simulink model "DISCON_NREL5MW_update"  (R2020b)
settings: Solver=FixedStepDiscrete  StartTime=0.0  StopTime=inf  FixedStep=Control.DT  RelTol=1e-3
values from neighbouring files (symbols this model uses):
  Gd_Fwave = c2d(Sys{OperatingPoint}('omega_r','F_{hydro}'),Control.TimeStep,'tustin')    [ControlParams_NREL5MW.m]
  Gd_Mwave = c2d(Sys{OperatingPoint}('omega_r','M_{hydro}'),Control.TimeStep,'tustin')    [ControlParams_NREL5MW.m]
  InvGp = inv(Gp)    [ControlParams_NREL5MW.m]
  Kff_gain = 0.3    [InitCompDISCON.m]
undefined symbols (not defined in the file or in its folder): CertificationSettings, Control, DelTFd, DiscIntNeverNeededParam, Drivetrain, Freq_Mixing, P_InitAngle
settings Model: Creator=evansolingen  LastModifiedBy=ahegazy
settings DataIOCC: LimitDataPoints=on  SaveFormat=Array  SignalLoggingSaveFormat=ModelDataLogs  SaveOutput=off  SignalLogging=off  SaveTime=off  ReturnWorkspaceOutputs=off
settings OptimizationCC: ExpressionDepthLimit=2147483647  LifeSpan=inf
settings DebuggingCC: UnderspecifiedInitializationDetection=Classic  MergeDetectMultiDrivingBlocksExec=none  SolverPrmCheckMsg=warning  MultiTaskDSMMsg=warning  MultiTaskCondExecSysMsg=none  FcnCallInpInsideContextMsg=warning  AllowSymbolicDim=off  StateNameClashWarn=warning  SFUnexpectedBacktrackingDiag=warning  SFNoUnconditionalDefaultTransitionDiag=warning  SFExecutionAtInitializationDiag=none  ArithmeticOperatorsInVariantConditions=warning
settings HardwareCC: ProdBitPerPointer=32  ProdBitPerSizeT=32  ProdBitPerPtrDiffT=32  ProdLargestAtomicFloat=None  ProdIntDivRoundTo=Undefined  ProdEndianess=Unspecified  ProdWordSize=32  ProdHWDeviceType=32-bit Generic
settings ModelReferenceCC: UpdateModelReferenceTargets=Force  PropagateSignalLabelsOutOfModel=off
settings SFSimCC: SimUseLocalCustomCode=off  SimParseCustomCode=off  CustomCodeUndefinedFunction=UseInterfaceOnly
settings RTWCC: Description=DISCON DLL Target (for use with GH BLADED)  SystemTargetFile=discon.tlc  TemplateMakefile=discon_vc.tmf  RTWUseLocalCustomCode=off
settings CodeAppCC: StateflowObjectComments=on
settings GRTTargetCC: TargetLangStandard=C89/C90 (ANSI)  CombineOutputUpdateFcns=off  GRTInterface=on  UseToolchainInfoCompliant=off  ExtModeMexFile=noextcomm
settings ConfigComp: CovMetricSettings=dw  CovSaveCumulativeToWorkspaceVar=on  CovSaveSingleToWorkspaceVar=on  CovExternalEMLEnable=off

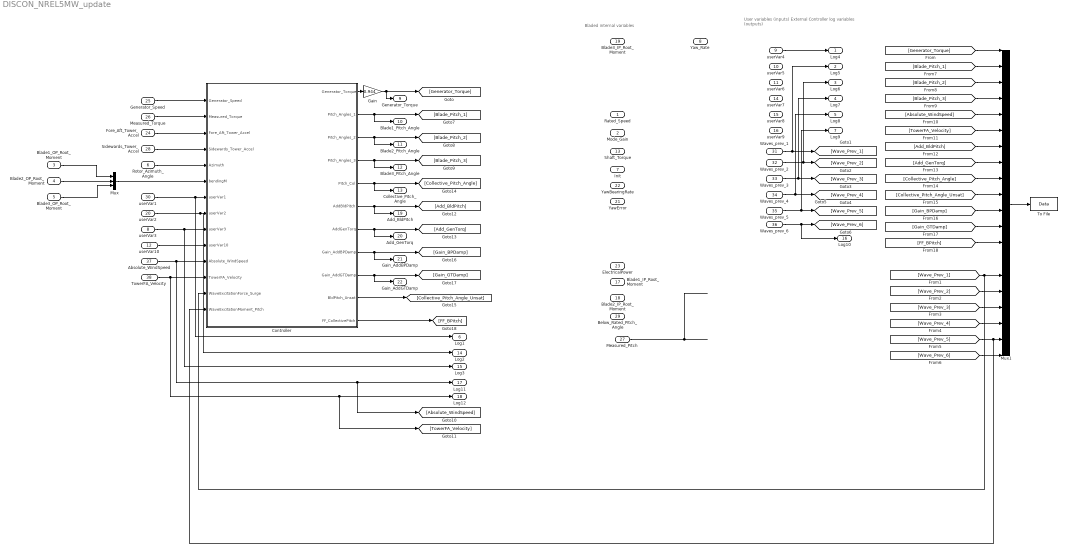
== system DISCON_NREL5MW_update ==
  note: Bladed internal variables
  note: User variables (inputs)
      | External Controller log variables (outputs)
  Rated_Speed : Inport  PortDimensions=1
  Mode_Gain : Inport  Port=2  PortDimensions=1
  Blade1_OP_Root_Moment : Inport  Port=3  PortDimensions=1
  Blade2_OP_Root_Moment : Inport  Port=4  PortDimensions=1
  Blade3_OP_Root_Moment : Inport  Port=5  PortDimensions=1
  Rotor_Azimuth_Angle : Inport  Port=6  PortDimensions=1
  Init : Inport  Port=7  PortDimensions=1
  userVar3 : Inport  Port=8  PortDimensions=1
  userVar4 : Inport  Port=9  PortDimensions=1
  userVar5 : Inport  Port=10  PortDimensions=1
  userVar6 : Inport  Port=11  PortDimensions=1
  userVar10 : Inport  Port=12  PortDimensions=1
  Shaft_Torque : Inport  Port=13  PortDimensions=1
  userVar7 : Inport  Port=14  PortDimensions=1
  userVar8 : Inport  Port=15  PortDimensions=1
  userVar9 : Inport  Port=16  PortDimensions=1
  Blade1_IP_Root_Moment : Inport  Port=17  PortDimensions=1
  Blade2_IP_Root_Moment : Inport  Port=18  PortDimensions=1
  Blade3_IP_Root_Moment : Inport  Port=19  PortDimensions=1
  userVar2 : Inport  Port=20  PortDimensions=1
  YawError : Inport  Port=21  PortDimensions=1
  YawBearingRate : Inport  Port=22  PortDimensions=1
  ElectricalPower : Inport  Port=23  PortDimensions=1
  Fore_Aft_Tower_Accel : Inport  Port=24  PortDimensions=1
  Generator_Speed : Inport  Port=25  PortDimensions=1
  Measured_Torque : Inport  Port=26  PortDimensions=1
  Measured_Pitch : Inport  Port=27  PortDimensions=1
  Sidewards_Tower_Accel : Inport  Port=28  PortDimensions=1
  Below_Rated_Pitch_Angle : Inport  Port=29  PortDimensions=1
  userVar1 : Inport  Port=30  PortDimensions=1
  Waves_prev_1 : Inport  Port=31  PortDimensions=1
  Waves_prev_2 : Inport  Port=32  PortDimensions=1
  Waves_prev_3 : Inport  Port=33  PortDimensions=1
  Waves_prev_4 : Inport  Port=34  PortDimensions=1
  Waves_prev_5 : Inport  Port=35  PortDimensions=1
  Waves_prev_6 : Inport  Port=36  PortDimensions=1
  Absolute_WindSpeed : Inport  Port=37  PortDimensions=1
  TowerFA_Velocity : Inport  Port=38  PortDimensions=1
  Controller : Subsystem
  Gain : Gain  Gain=0.944
  Mux : Mux  Inputs=3
  Mux1 : Mux  Inputs=20
  To File : ToFile  Filename=Data  MatrixName=Data
  Log4 : Outport  PortDimensions=1  VectorParamsAs1DForOutWhenUnconnected=off
  Log5 : Outport  Port=2  PortDimensions=1  VectorParamsAs1DForOutWhenUnconnected=off
  Log6 : Outport  Port=3  PortDimensions=1  VectorParamsAs1DForOutWhenUnconnected=off
  Log7 : Outport  Port=4  PortDimensions=1  VectorParamsAs1DForOutWhenUnconnected=off
  Log8 : Outport  Port=5  PortDimensions=1  VectorParamsAs1DForOutWhenUnconnected=off
  Log1 : Outport  Port=6  PortDimensions=1  VectorParamsAs1DForOutWhenUnconnected=off
  Log9 : Outport  Port=7  PortDimensions=1  VectorParamsAs1DForOutWhenUnconnected=off
  Yaw_Rate : Outport  Port=8  PortDimensions=1  VectorParamsAs1DForOutWhenUnconnected=off
  Generator_Torque : Outport  Port=9  PortDimensions=1  VectorParamsAs1DForOutWhenUnconnected=off
  Blade1_Pitch_Angle : Outport  Port=10  PortDimensions=1  VectorParamsAs1DForOutWhenUnconnected=off
  Blade2_Pitch_Angle : Outport  Port=11  PortDimensions=1  VectorParamsAs1DForOutWhenUnconnected=off
  Blade3_Pitch_Angle : Outport  Port=12  PortDimensions=1  VectorParamsAs1DForOutWhenUnconnected=off
  Collective_Pitch_Angle : Outport  Port=13  PortDimensions=1  VectorParamsAs1DForOutWhenUnconnected=off
  Log2 : Outport  Port=14  PortDimensions=1  VectorParamsAs1DForOutWhenUnconnected=off
  Log3 : Outport  Port=15  PortDimensions=1  VectorParamsAs1DForOutWhenUnconnected=off
  Log10 : Outport  Port=16  PortDimensions=1  VectorParamsAs1DForOutWhenUnconnected=off
  Log11 : Outport  Port=17  PortDimensions=1  VectorParamsAs1DForOutWhenUnconnected=off
  Log12 : Outport  Port=18  PortDimensions=1  VectorParamsAs1DForOutWhenUnconnected=off
  Add_BldPitch : Outport  Port=19  PortDimensions=1  VectorParamsAs1DForOutWhenUnconnected=off
  Add_GenTorq : Outport  Port=20  PortDimensions=1  VectorParamsAs1DForOutWhenUnconnected=off
  Gain_AddBPDamp : Outport  Port=21  PortDimensions=1  VectorParamsAs1DForOutWhenUnconnected=off
  Gain_AddGTDamp : Outport  Port=22  PortDimensions=1  VectorParamsAs1DForOutWhenUnconnected=off
  wires:
  Fore_Aft_Tower_Accel/1 -> Controller/3(Fore_Aft_Tower_Accel)
  Measured_Pitch/1 -> ?
  Generator_Speed/1 -> Controller/1(Generator_Speed)
  Controller/1(Generator_Torque) -> Gain/1
  userVar3/1 -> Log3/1, Controller/9(userVar3)
  userVar4/1 -> Log4/1
  Gain/1 -> [Generator_Torque], Generator_Torque/1
  Measured_Torque/1 -> Controller/2(Measured_Torque)
  Sidewards_Tower_Accel/1 -> Controller/4(Sidewards_Tower_Accel)
  Rotor_Azimuth_Angle/1 -> Controller/5(Azimuth)
  Blade1_OP_Root_Moment/1 -> Mux/1
  Blade2_OP_Root_Moment/1 -> Mux/2
  Blade3_OP_Root_Moment/1 -> Mux/3
  Mux/1 -> Controller/6(bendingM)
  Controller/2(Pitch_Angles_1) -> Blade1_Pitch_Angle/1, [Blade_Pitch_1]
  Controller/3(Pitch_Angles_2) -> Blade2_Pitch_Angle/1, [Blade_Pitch_2]
  Controller/4(Pitch_Angles_3) -> Blade3_Pitch_Angle/1, [Blade_Pitch_3]
  Controller/5(Pitch_Col) -> [Collective_Pitch_Angle], Collective_Pitch_Angle/1
  userVar1/1 -> Log1/1, Controller/7(userVar1)
  userVar2/1 -> Log2/1, Controller/8(userVar2)
  userVar10/1 -> Controller/10(userVar10)
  Mux1/1 -> To File/1
  [Generator_Torque] -> Mux1/1
  Waves_prev_1/1 -> Log5/1, [Wave_Prev_1]
  Waves_prev_2/1 -> Log6/1, [Wave_Prev_2]
  Waves_prev_3/1 -> Log7/1, [Wave_Prev_3]
  Waves_prev_4/1 -> Log8/1, [Wave_Prev_4]
  Waves_prev_5/1 -> Log9/1, [Wave_Prev_5]
  Waves_prev_6/1 -> Log10/1, [Wave_Prev_6]
  [Wave_Prev_6] -> Mux1/20
  [Wave_Prev_5] -> Controller/14(WaveExcitationMoment_Pitch), Mux1/19
  [Wave_Prev_4] -> Mux1/18
  [Wave_Prev_3] -> Mux1/17
  [Wave_Prev_2] -> Mux1/16
  [Wave_Prev_1] -> Mux1/15, Controller/13(WaveExcitationForce_Surge)
  [Blade_Pitch_1] -> Mux1/2
  [Blade_Pitch_2] -> Mux1/3
  [Blade_Pitch_3] -> Mux1/4
  TowerFA_Velocity/1 -> Controller/12(TowerFA_Velocity), [TowerFA_Velocity], Log12/1
  [Absolute_WindSpeed] -> Mux1/5
  [TowerFA_Velocity] -> Mux1/6
  [Add_BldPitch] -> Mux1/7
  [Add_GenTorq] -> Mux1/8
  Absolute_WindSpeed/1 -> [Absolute_WindSpeed], Log11/1, Controller/11(Absolute_WindSpeed)
  Controller/6(AddBldPitch) -> Add_BldPitch/1, [Add_BldPitch]
  Controller/7(AddGenTorq) -> Add_GenTorq/1, [Add_GenTorq]
  Controller/8(Gain_AddBPDamp) -> Gain_AddBPDamp/1, [Gain_BPDamp]
  Controller/9(Gain_AddGTDamp) -> Gain_AddGTDamp/1, [Gain_GTDamp]
  [Collective_Pitch_Angle] -> Mux1/9
  Controller/10(BldPitch_Unsat) -> [Collective_Pitch_Angle_Unsat]
  [Collective_Pitch_Angle_Unsat] -> Mux1/10
  [Gain_BPDamp] -> Mux1/11
  [Gain_GTDamp] -> Mux1/12
  [FF_BPitch] -> Mux1/13
  Controller/11(FF_CollectivePitch) -> [FF_BPitch]

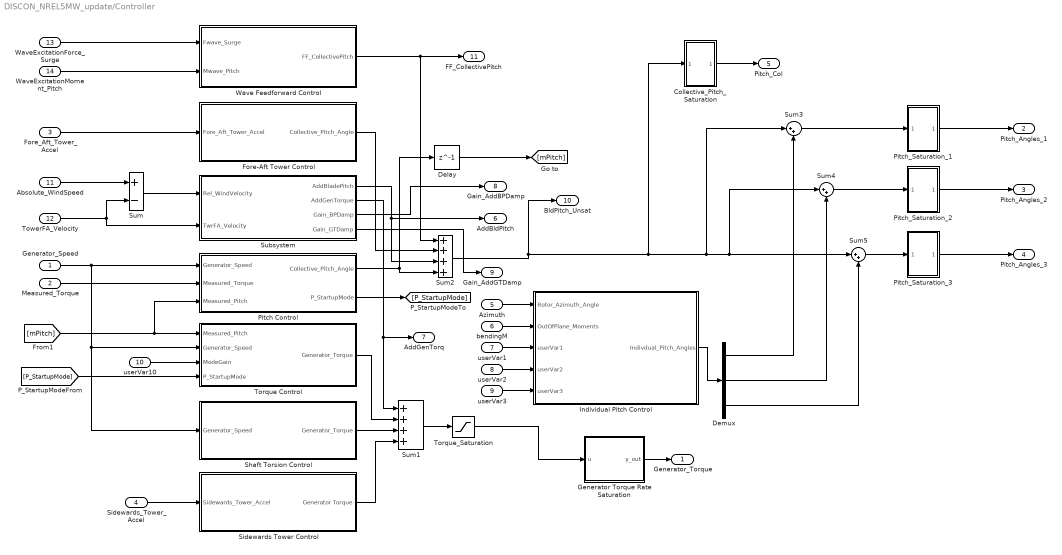
== system DISCON_NREL5MW_update/Controller ==
  Generator_Speed : Inport
  Measured_Torque : Inport  Port=2
  Fore_Aft_Tower_Accel : Inport  Port=3
  Sidewards_Tower_Accel : Inport  Port=4  PortDimensions=1
  Azimuth : Inport  Port=5  PortDimensions=1
  bendingM : Inport  Port=6
  userVar1 : Inport  Port=7  PortDimensions=1
  userVar2 : Inport  Port=8  PortDimensions=1
  userVar3 : Inport  Port=9  PortDimensions=1
  userVar10 : Inport  Port=10  PortDimensions=1
  Absolute_WindSpeed : Inport  Port=11  PortDimensions=1
  TowerFA_Velocity : Inport  Port=12  PortDimensions=1
  WaveExcitationForce_Surge : Inport  Port=13
  WaveExcitationMoment_Pitch : Inport  Port=14
  Collective_Pitch_Saturation : Subsystem
  Delay : Delay  DelayLength=1
  Demux : Demux  Outputs=3
  Fore-Aft Tower Control : Subsystem
  Generator Torque Rate Saturation : Subsystem
  Individual Pitch Control : Subsystem
  Pitch Control : Subsystem
  Pitch_Saturation_1 : Subsystem
  Pitch_Saturation_2 : Subsystem
  Pitch_Saturation_3 : Subsystem
  Shaft Torsion Control : Subsystem
  Sidewards Tower Control : Subsystem
  Subsystem : Subsystem
  Sum : Sum  Inputs=+-
  Sum1 : Sum  Inputs=++++
  Sum2 : Sum  Inputs=++++
  Sum3 : Sum  Inputs=|++
  Sum4 : Sum  Inputs=|++
  Sum5 : Sum  Inputs=|++
  Torque Control : Subsystem
  Torque_Saturation : Saturate  UpperLimit=Control.Torque.Limit  LowerLimit=Control.Torque.Min
  Wave Feedforward Control : Subsystem
  Generator_Torque : Outport  VectorParamsAs1DForOutWhenUnconnected=off
  Pitch_Angles_1 : Outport  Port=2  PortDimensions=1  VectorParamsAs1DForOutWhenUnconnected=off
  Pitch_Angles_2 : Outport  Port=3  PortDimensions=1  VectorParamsAs1DForOutWhenUnconnected=off
  Pitch_Angles_3 : Outport  Port=4  PortDimensions=1  VectorParamsAs1DForOutWhenUnconnected=off
  Pitch_Col : Outport  Port=5  PortDimensions=1  VectorParamsAs1DForOutWhenUnconnected=off
  AddBldPitch : Outport  Port=6  PortDimensions=1  VectorParamsAs1DForOutWhenUnconnected=off
  AddGenTorq : Outport  Port=7  PortDimensions=1  VectorParamsAs1DForOutWhenUnconnected=off
  Gain_AddBPDamp : Outport  Port=8  PortDimensions=1  VectorParamsAs1DForOutWhenUnconnected=off
  Gain_AddGTDamp : Outport  Port=9  PortDimensions=1  VectorParamsAs1DForOutWhenUnconnected=off
  BldPitch_Unsat : Outport  Port=10  PortDimensions=1  VectorParamsAs1DForOutWhenUnconnected=off
  FF_CollectivePitch : Outport  Port=11
  wires:
  Sidewards_Tower_Accel/1 -> Sidewards Tower Control/1(Sidewards_Tower_Accel)
  Fore_Aft_Tower_Accel/1 -> Fore-Aft Tower Control/1(Fore_Aft_Tower_Accel)
  Fore-Aft Tower Control/1(Collective_Pitch_Angle) -> Sum2/2
  Torque Control/1(Generator_Torque) -> Sum1/2
  Sidewards Tower Control/1(Generator Torque) -> Sum1/4
  Measured_Torque/1 -> Pitch Control/2(Measured_Torque)
  Shaft Torsion Control/1(Generator_Torque) -> Sum1/3
  userVar10/1 -> Torque Control/3(ModeGain)
  Sum1/1 -> Torque_Saturation/1
  Pitch_Saturation_1/1(y_out) -> Pitch_Angles_1/1
  Generator_Speed/1 -> Torque Control/2(Generator_Speed), Shaft Torsion Control/1(Generator_Speed), Pitch Control/1(Generator_Speed)
  [P_StartupMode] -> Torque Control/4(P_StartupMode)
  Pitch Control/2(P_StartupMode) -> [P_StartupMode]
  Pitch Control/1(Collective_Pitch_Angle) -> Delay/1, Sum2/4
  Pitch_Saturation_2/1(y_out) -> Pitch_Angles_2/1
  Pitch_Saturation_3/1(y_out) -> Pitch_Angles_3/1
  Individual Pitch Control/1(Indivdual_Pitch_Angles) -> Demux/1
  bendingM/1 -> Individual Pitch Control/2(OutOfPlane_Moments)
  Azimuth/1 -> Individual Pitch Control/1(Rotor_Azimuth_Angle)
  Sum3/1 -> Pitch_Saturation_1/1(In1)
  Sum4/1 -> Pitch_Saturation_2/1(In1)
  Sum5/1 -> Pitch_Saturation_3/1(In1)
  Sum2/1 -> Collective_Pitch_Saturation/1(In1), Sum4/1, Sum5/1, Sum3/1, BldPitch_Unsat/1
  Delay/1 -> [mPitch]
  Demux/1 -> Sum3/2
  Demux/2 -> Sum4/2
  Demux/3 -> Sum5/2
  [mPitch] -> Pitch Control/3(Measured_Pitch), Torque Control/1(Measured_Pitch)
  userVar1/1 -> Individual Pitch Control/3(userVar1)
  userVar2/1 -> Individual Pitch Control/4(userVar2)
  userVar3/1 -> Individual Pitch Control/5(userVar3)
  Absolute_WindSpeed/1 -> Sum/1
  TowerFA_Velocity/1 -> Subsystem/2(TwrFA_Velocity), Sum/2
  Subsystem/1(AddBladePitch) -> Sum2/3, AddBldPitch/1
  Subsystem/2(AddGenTorque) -> AddGenTorq/1, Sum1/1
  Sum/1 -> Subsystem/1(Rel_WindVelocity)
  Subsystem/3(Gain_BPDamp) -> Gain_AddBPDamp/1
  Subsystem/4(Gain_GTDamp) -> Gain_AddGTDamp/1
  Collective_Pitch_Saturation/1(y_out) -> Pitch_Col/1
  Wave Feedforward Control/1(FF_CollectivePitch) -> FF_CollectivePitch/1, Sum2/1
  WaveExcitationForce_Surge/1 -> Wave Feedforward Control/1(Fwave_Surge)
  WaveExcitationMoment_Pitch/1 -> Wave Feedforward Control/2(Mwave_Pitch)
  Torque_Saturation/1 -> Generator Torque Rate Saturation/1(u)
  Generator Torque Rate Saturation/1(y_out) -> Generator_Torque/1

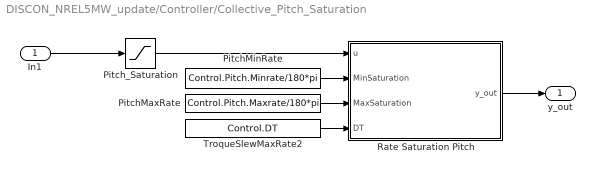
== system DISCON_NREL5MW_update/Controller/Collective_Pitch_Saturation ==
  In1 : Inport
  PitchMaxRate : Constant  Value=Control.Pitch.Maxrate/180*pi
  PitchMinRate : Constant  Value=Control.Pitch.Minrate/180*pi
  Pitch_Saturation : Saturate  UpperLimit=Control.Pitch.Max*pi/180  LowerLimit=Control.Pitch.Min*pi/180
  Rate Saturation Pitch : MATLAB Function  TreatAsAtomicUnit=on
  TroqueSlewMaxRate2 : Constant  Value=Control.DT
  y_out : Outport
  wires:
  Pitch_Saturation/1 -> Rate Saturation Pitch/1(u)
  PitchMinRate/1 -> Rate Saturation Pitch/2(MinSaturation)
  In1/1 -> Pitch_Saturation/1
  TroqueSlewMaxRate2/1 -> Rate Saturation Pitch/4(DT)
  PitchMaxRate/1 -> Rate Saturation Pitch/3(MaxSaturation)
  Rate Saturation Pitch/1(y_out) -> y_out/1

== system DISCON_NREL5MW_update/Controller/Fore-Aft Tower Control ==
  note: Fore-Aft tower damping
  Fore_Aft_Tower_Accel : Inport
  Discrete-Time Integrator : DiscreteIntegrator  SampleTime=-1  ICPrevOutput=DiscIntNeverNeededParam  ICPrevScaledInput=DiscIntNeverNeededParam
  Gain : Gain  Gain=Control.ForeAft.Gain
  Pitch_Saturation : Saturate  UpperLimit=Control.ForeAft.MaxPitchAmplitude*pi/180  LowerLimit=-Control.ForeAft.MaxPitchAmplitude*pi/180
  Collective_Pitch_Angle : Outport  VectorParamsAs1DForOutWhenUnconnected=off
  wires:
  Fore_Aft_Tower_Accel/1 -> Discrete-Time Integrator/1
  Pitch_Saturation/1 -> Collective_Pitch_Angle/1
  Discrete-Time Integrator/1 -> Gain/1
  Gain/1 -> Pitch_Saturation/1

== system DISCON_NREL5MW_update/Controller/Generator Torque Rate Saturation ==
  u : Inport
  Rate Saturation Torque : MATLAB Function  TreatAsAtomicUnit=on
  TroqueSlewMaxRate : Constant  Value=Control.Torque.Slewrate
  TroqueSlewMaxRate1 : Constant  Value=Control.DT
  TroqueSlewMinRate : Constant  Value=-Control.Torque.Slewrate
  y_out : Outport
  wires:
  TroqueSlewMaxRate/1 -> Rate Saturation Torque/3(MaxSaturation)
  TroqueSlewMaxRate1/1 -> Rate Saturation Torque/4(DT)
  TroqueSlewMinRate/1 -> Rate Saturation Torque/2(MinSaturation)
  u/1 -> Rate Saturation Torque/1(u)
  Rate Saturation Torque/1(y_out) -> y_out/1

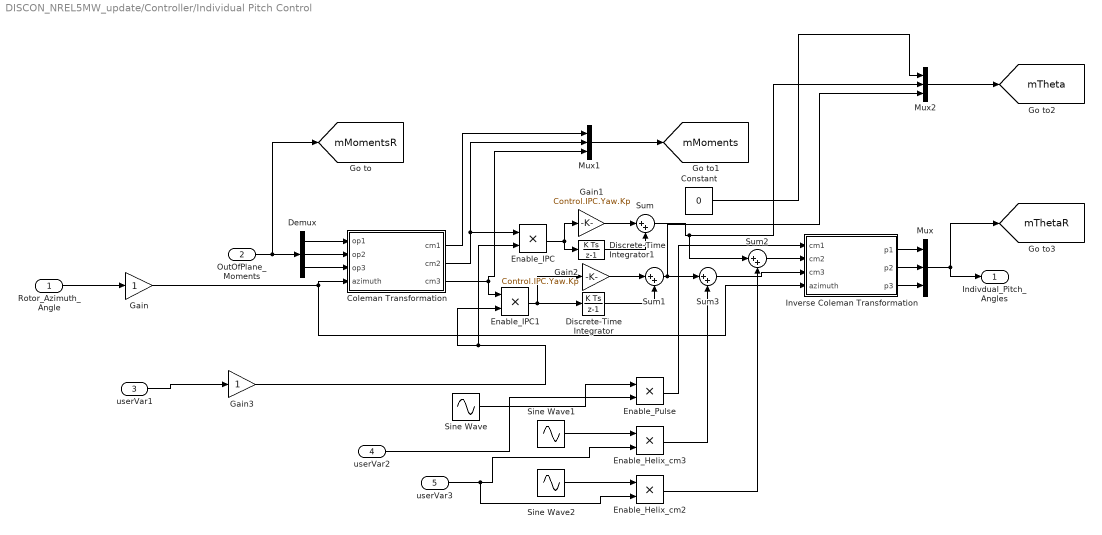
== system DISCON_NREL5MW_update/Controller/Individual Pitch Control ==
  Rotor_Azimuth_Angle : Inport
  OutOfPlane_Moments : Inport  Port=2
  userVar1 : Inport  Port=3  PortDimensions=1
  userVar2 : Inport  Port=4  PortDimensions=1
  userVar3 : Inport  Port=5  PortDimensions=1
  Coleman Transformation : Subsystem
  Constant : Constant  Value=0
  Demux : Demux  Outputs=3
  Discrete-Time Integrator : DiscreteIntegrator  gainval=Control.IPC.Yaw.Ki+1e-20  SampleTime=-1  ICPrevOutput=DiscIntNeverNeededParam  ICPrevScaledInput=DiscIntNeverNeededParam
  Discrete-Time Integrator1 : DiscreteIntegrator  gainval=Control.IPC.Yaw.Ki+1e-20  SampleTime=-1  ICPrevOutput=DiscIntNeverNeededParam  ICPrevScaledInput=DiscIntNeverNeededParam
  Enable_Helix_cm2 : Product  Inputs=**
  Enable_Helix_cm3 : Product  Inputs=**
  Enable_IPC : Product  Inputs=**
  Enable_IPC1 : Product  Inputs=**
  Enable_Pulse : Product  Inputs=**
  Gain : Gain
  Gain1 : Gain  Gain=Control.IPC.Yaw.Kp
  Gain2 : Gain  Gain=Control.IPC.Yaw.Kp
  Gain3 : Gain
  Inverse Coleman Transformation : Subsystem
  Mux : Mux  Inputs=3
  Mux1 : Mux  Inputs=3
  Mux2 : Mux  Inputs=3
  Sine Wave : Sin  Frequency=Freq_Mixing  Phase=-pi  SampleTime=0
  Sine Wave1 : Sin  Frequency=Freq_Mixing  Phase=-pi  SampleTime=0
  Sine Wave2 : Sin  Frequency=Freq_Mixing  Phase=-1/2*pi  SampleTime=0
  Sum{,1..3} (4 alike) : Sum  Inputs=|++
  Indivdual_Pitch_Angles : Outport
  tag scope: mMoments=global, mMomentsR=global, mTheta=global, mThetaR=global
  wires:
  Mux/1 -> Indivdual_Pitch_Angles/1, [mThetaR]
  Inverse Coleman Transformation/1(p1) -> Mux/1
  Inverse Coleman Transformation/2(p2) -> Mux/2
  Inverse Coleman Transformation/3(p3) -> Mux/3
  Demux/1 -> Coleman Transformation/1(op1)
  Demux/2 -> Coleman Transformation/2(op2)
  Demux/3 -> Coleman Transformation/3(op3)
  OutOfPlane_Moments/1 -> [mMomentsR], Demux/1
  Rotor_Azimuth_Angle/1 -> Gain/1
  Coleman Transformation/1(cm1) -> Mux1/1
  Coleman Transformation/2(cm2) -> Mux1/2, Enable_IPC/1
  Coleman Transformation/3(cm3) -> Mux1/3, Enable_IPC1/1
  Mux1/1 -> [mMoments]
  Gain/1 -> Inverse Coleman Transformation/4(azimuth), Coleman Transformation/4(azimuth)
  Discrete-Time Integrator1/1 -> Sum/2
  Gain1/1 -> Sum/1
  Discrete-Time Integrator/1 -> Sum1/2
  Gain2/1 -> Sum1/1
  Enable_IPC/1 -> Discrete-Time Integrator1/1, Gain1/1
  Enable_IPC1/1 -> Gain2/1, Discrete-Time Integrator/1
  Sum1/1 -> Mux2/3, Sum3/1
  Sum/1 -> Sum2/1, Mux2/2
  Constant/1 -> Mux2/1
  Mux2/1 -> [mTheta]
  userVar1/1 -> Gain3/1
  Gain3/1 -> Enable_IPC1/2, Enable_IPC/2
  Sum2/1 -> Inverse Coleman Transformation/2(cm2)
  Sum3/1 -> Inverse Coleman Transformation/3(cm3)
  Enable_Pulse/1 -> Inverse Coleman Transformation/1(cm1)
  Enable_Helix_cm3/1 -> Sum3/2
  Enable_Helix_cm2/1 -> Sum2/2
  Sine Wave/1 -> Enable_Pulse/1
  Sine Wave1/1 -> Enable_Helix_cm3/1
  Sine Wave2/1 -> Enable_Helix_cm2/1
  userVar2/1 -> Enable_Pulse/2
  userVar3/1 -> Enable_Helix_cm2/2, Enable_Helix_cm3/2

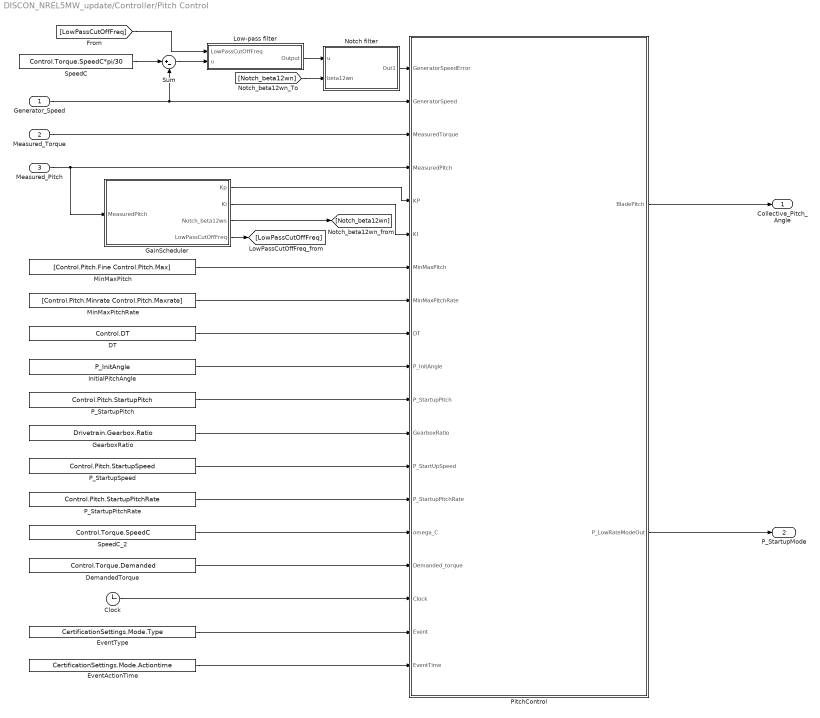
== system DISCON_NREL5MW_update/Controller/Pitch Control ==
  Generator_Speed : Inport
  Measured_Torque : Inport  Port=2
  Measured_Pitch : Inport  Port=3
  Clock : Clock
  DT : Constant  Value=Control.DT
  DemandedTorque : Constant  Value=Control.Torque.Demanded
  EventActionTime : Constant  Value=CertificationSettings.Mode.Actiontime
  EventType : Constant  Value=CertificationSettings.Mode.Type
  GainScheduler : Subsystem
  GearboxRatio : Constant  Value=Drivetrain.Gearbox.Ratio
  InitialPitchAngle : Constant  Value=P_InitAngle
  Low-pass filter : Subsystem
  MinMaxPitch : Constant  Value=[Control.Pitch.Fine Control.Pitch.Max]
  MinMaxPitchRate : Constant  Value=[Control.Pitch.Minrate Control.Pitch.Maxrate]
  Notch filter : Subsystem
  P_StartupPitch : Constant  Value=Control.Pitch.StartupPitch
  P_StartupPitchRate : Constant  Value=Control.Pitch.StartupPitchRate
  P_StartupSpeed : Constant  Value=Control.Pitch.StartupSpeed
  PitchControl : MATLAB Function  TreatAsAtomicUnit=on
  SpeedC : Constant  Value=Control.Torque.SpeedC*pi/30
  SpeedC_2 : Constant  Value=Control.Torque.SpeedC
  Sum : Sum  Inputs=|+-
  Collective_Pitch_Angle : Outport  VectorParamsAs1DForOutWhenUnconnected=off
  P_StartupMode : Outport  Port=2  VectorParamsAs1DForOutWhenUnconnected=off
  wires:
  MinMaxPitch/1 -> PitchControl/7(MinMaxPitch)
  MinMaxPitchRate/1 -> PitchControl/8(MinMaxPitchRate)
  PitchControl/1(BladePitch) -> Collective_Pitch_Angle/1
  Measured_Torque/1 -> PitchControl/3(MeasuredTorque)
  SpeedC/1 -> Sum/1
  Generator_Speed/1 -> PitchControl/2(GeneratorSpeed), Sum/2
  Sum/1 -> Low-pass filter/2(u)
  PitchControl/2(P_LowRateModeOut) -> P_StartupMode/1
  DT/1 -> PitchControl/9(DT)
  P_StartupPitch/1 -> PitchControl/11(P_StartupPitch)
  InitialPitchAngle/1 -> PitchControl/10(P_InitAngle)
  GearboxRatio/1 -> PitchControl/12(GearboxRatio)
  P_StartupSpeed/1 -> PitchControl/13(P_StartUpSpeed)
  P_StartupPitchRate/1 -> PitchControl/14(P_StartupPitchRate)
  SpeedC_2/1 -> PitchControl/15(omega_C)
  DemandedTorque/1 -> PitchControl/16(Demanded_torque)
  Measured_Pitch/1 -> GainScheduler/1(MeasuredPitch), PitchControl/4(MeasuredPitch)
  EventType/1 -> PitchControl/18(Event)
  Clock/1 -> PitchControl/17(Clock)
  EventActionTime/1 -> PitchControl/19(EventTime)
  GainScheduler/1(Kp) -> PitchControl/5(KP)
  GainScheduler/2(Ki) -> PitchControl/6(KI)
  [Notch_beta12wn] -> Notch filter/2(beta12wn)
  GainScheduler/3(Notch_beta12wn) -> [Notch_beta12wn]
  Low-pass filter/1(Output) -> Notch filter/1(u)
  Notch filter/1(Out1) -> PitchControl/1(GeneratorSpeedError)
  GainScheduler/4(LowPassCutOffFreq) -> [LowPassCutOffFreq]
  [LowPassCutOffFreq] -> Low-pass filter/1(LowPassCutOffFreq)

== system DISCON_NREL5MW_update/Controller/Pitch_Saturation_1 ==
  In1 : Inport
  PitchMaxRate : Constant  Value=Control.Pitch.Maxrate/180*pi
  PitchMinRate : Constant  Value=Control.Pitch.Minrate/180*pi
  Pitch_Saturation : Saturate  UpperLimit=Control.Pitch.Max*pi/180  LowerLimit=Control.Pitch.Min*pi/180
  Rate Saturation Pitch : MATLAB Function  TreatAsAtomicUnit=on
  TroqueSlewMaxRate2 : Constant  Value=Control.DT
  y_out : Outport
  wires:
  Pitch_Saturation/1 -> Rate Saturation Pitch/1(u)
  PitchMinRate/1 -> Rate Saturation Pitch/2(MinSaturation)
  In1/1 -> Pitch_Saturation/1
  TroqueSlewMaxRate2/1 -> Rate Saturation Pitch/4(DT)
  PitchMaxRate/1 -> Rate Saturation Pitch/3(MaxSaturation)
  Rate Saturation Pitch/1(y_out) -> y_out/1

== system DISCON_NREL5MW_update/Controller/Pitch_Saturation_2 ==
  In1 : Inport
  PitchMaxRate : Constant  Value=Control.Pitch.Maxrate/180*pi
  PitchMinRate : Constant  Value=Control.Pitch.Minrate/180*pi
  Pitch_Saturation : Saturate  UpperLimit=Control.Pitch.Max*pi/180  LowerLimit=Control.Pitch.Min*pi/180
  Rate Saturation Pitch : MATLAB Function  TreatAsAtomicUnit=on
  TroqueSlewMaxRate2 : Constant  Value=Control.DT
  y_out : Outport
  wires:
  Pitch_Saturation/1 -> Rate Saturation Pitch/1(u)
  PitchMinRate/1 -> Rate Saturation Pitch/2(MinSaturation)
  In1/1 -> Pitch_Saturation/1
  TroqueSlewMaxRate2/1 -> Rate Saturation Pitch/4(DT)
  PitchMaxRate/1 -> Rate Saturation Pitch/3(MaxSaturation)
  Rate Saturation Pitch/1(y_out) -> y_out/1

== system DISCON_NREL5MW_update/Controller/Pitch_Saturation_3 ==
  In1 : Inport
  PitchMaxRate : Constant  Value=Control.Pitch.Maxrate/180*pi
  PitchMinRate : Constant  Value=Control.Pitch.Minrate/180*pi
  Pitch_Saturation : Saturate  UpperLimit=Control.Pitch.Max*pi/180  LowerLimit=Control.Pitch.Min*pi/180
  Rate Saturation Pitch : MATLAB Function  TreatAsAtomicUnit=on
  TroqueSlewMaxRate2 : Constant  Value=Control.DT
  y_out : Outport
  wires:
  Pitch_Saturation/1 -> Rate Saturation Pitch/1(u)
  PitchMinRate/1 -> Rate Saturation Pitch/2(MinSaturation)
  In1/1 -> Pitch_Saturation/1
  TroqueSlewMaxRate2/1 -> Rate Saturation Pitch/4(DT)
  PitchMaxRate/1 -> Rate Saturation Pitch/3(MaxSaturation)
  Rate Saturation Pitch/1(y_out) -> y_out/1

== system DISCON_NREL5MW_update/Controller/Shaft Torsion Control ==
  Generator_Speed : Inport
  Gain : Gain  Gain=0
  Generator_Torque : Outport  VectorParamsAs1DForOutWhenUnconnected=off
  wires:
  Generator_Speed/1 -> Gain/1
  Gain/1 -> Generator_Torque/1

== system DISCON_NREL5MW_update/Controller/Sidewards Tower Control ==
  Sidewards_Tower_Accel : Inport
  Gain : Gain  Gain=0
  Generator Torque : Outport  VectorParamsAs1DForOutWhenUnconnected=off
  wires:
  Sidewards_Tower_Accel/1 -> Gain/1
  Gain/1 -> Generator Torque/1

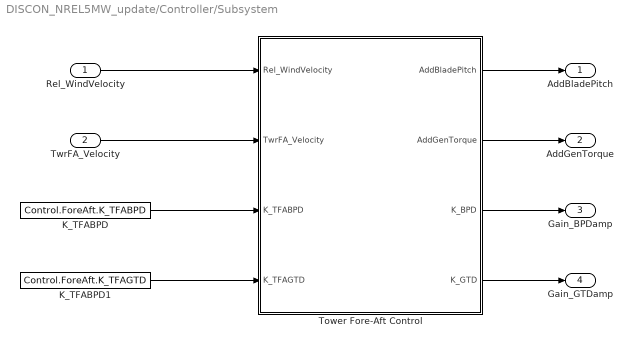
== system DISCON_NREL5MW_update/Controller/Subsystem ==
  Rel_WindVelocity : Inport
  TwrFA_Velocity : Inport  Port=2
  K_TFABPD : Constant  Value=Control.ForeAft.K_TFABPD
  K_TFABPD1 : Constant  Value=Control.ForeAft.K_TFAGTD
  Tower Fore-Aft Control : MATLAB Function  TreatAsAtomicUnit=on
  AddBladePitch : Outport
  AddGenTorque : Outport  Port=2
  Gain_BPDamp : Outport  Port=3
  Gain_GTDamp : Outport  Port=4
  wires:
  TwrFA_Velocity/1 -> Tower Fore-Aft Control/2(TwrFA_Velocity)
  K_TFABPD/1 -> Tower Fore-Aft Control/3(K_TFABPD)
  K_TFABPD1/1 -> Tower Fore-Aft Control/4(K_TFAGTD)
  Tower Fore-Aft Control/2(AddGenTorque) -> AddGenTorque/1
  Tower Fore-Aft Control/1(AddBladePitch) -> AddBladePitch/1
  Rel_WindVelocity/1 -> Tower Fore-Aft Control/1(Rel_WindVelocity)
  Tower Fore-Aft Control/3(K_BPD) -> Gain_BPDamp/1
  Tower Fore-Aft Control/4(K_GTD) -> Gain_GTDamp/1

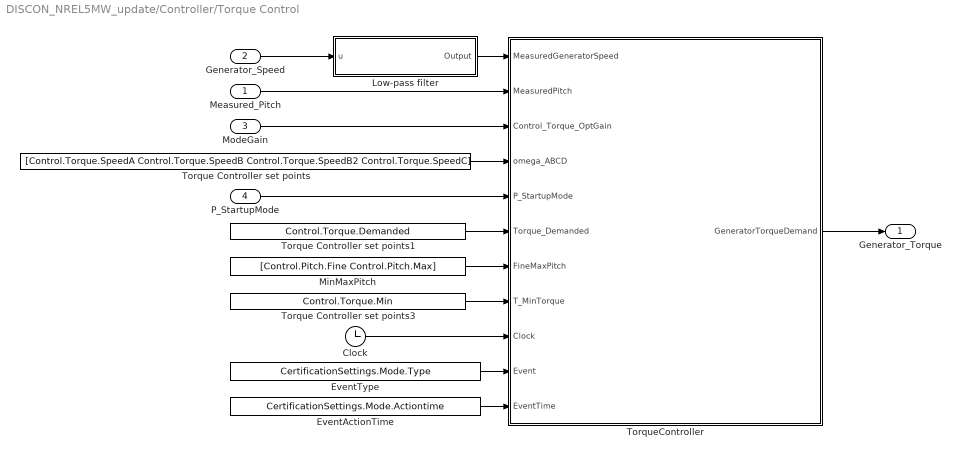
== system DISCON_NREL5MW_update/Controller/Torque Control ==
  Measured_Pitch : Inport
  Generator_Speed : Inport  Port=2
  ModeGain : Inport  Port=3
  P_StartupMode : Inport  Port=4
  Clock : Clock
  EventActionTime : Constant  Value=CertificationSettings.Mode.Actiontime
  EventType : Constant  Value=CertificationSettings.Mode.Type
  Low-pass filter : Subsystem
  MinMaxPitch : Constant  Value=[Control.Pitch.Fine Control.Pitch.Max]
  Torque Controller set points : Constant  Value=[Control.Torque.SpeedA Control.Torque.SpeedB Control.Torque.SpeedB2 Control.Torque.SpeedC]
  Torque Controller set points1 : Constant  Value=Control.Torque.Demanded
  Torque Controller set points3 : Constant  Value=Control.Torque.Min
  TorqueController : MATLAB Function  TreatAsAtomicUnit=on
  Generator_Torque : Outport  VectorParamsAs1DForOutWhenUnconnected=off
  wires:
  Generator_Speed/1 -> Low-pass filter/1(u)
  TorqueController/1(GeneratorTorqueDemand) -> Generator_Torque/1
  Measured_Pitch/1 -> TorqueController/2(MeasuredPitch)
  ModeGain/1 -> TorqueController/3(Control_Torque_OptGain)
  Torque Controller set points/1 -> TorqueController/4(omega_ABCD)
  P_StartupMode/1 -> TorqueController/5(P_StartupMode)
  Low-pass filter/1(Output) -> TorqueController/1(MeasuredGeneratorSpeed)
  Torque Controller set points3/1 -> TorqueController/8(T_MinTorque)
  MinMaxPitch/1 -> TorqueController/7(FineMaxPitch)
  Torque Controller set points1/1 -> TorqueController/6(Torque_Demanded)
  Clock/1 -> TorqueController/9(Clock)
  EventType/1 -> TorqueController/10(Event)
  EventActionTime/1 -> TorqueController/11(EventTime)

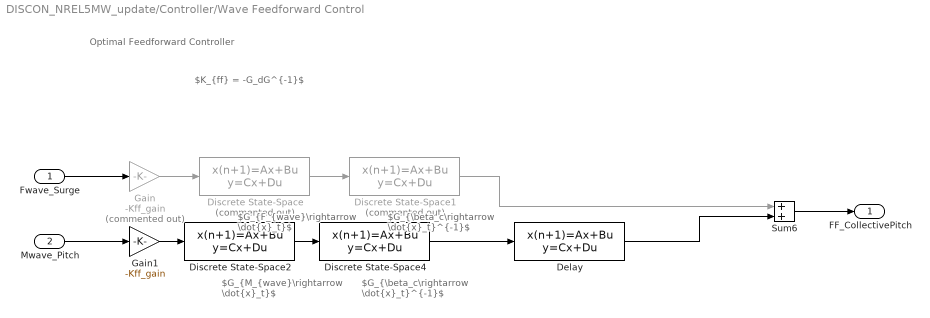
== system DISCON_NREL5MW_update/Controller/Wave Feedforward Control ==
  note: $K_{ff} = -G_dG^{-1}$
  note: Optimal Feedforward Controller
  note: $G_{F_{wave}\rightarrow \dot{x}_t}$
  note: $G_{M_{wave}\rightarrow \dot{x}_t}$
  note: $G_{\beta_c\rightarrow \dot{x}_t}^{-1}$
  note: $G_{\beta_c\rightarrow \dot{x}_t}^{-1}$
  Fwave_Surge : Inport
  Mwave_Pitch : Inport  Port=2
  Delay : DiscreteStateSpace  A=DelTFd.A  B=DelTFd.B  C=DelTFd.C  D=DelTFd.D  SampleTime=Control.DT
  Discrete State-Space : DiscreteStateSpace  Commented=on  A=Gd_Fwave.A  B=Gd_Fwave.B  C=Gd_Fwave.C  D=Gd_Fwave.D  SampleTime=Control.DT
  Discrete State-Space1 : DiscreteStateSpace  Commented=on  A=InvGp.A  B=InvGp.B  C=InvGp.C  D=InvGp.D  SampleTime=Control.DT
  Discrete State-Space2 : DiscreteStateSpace  A=Gd_Mwave.A  B=Gd_Mwave.B  C=Gd_Mwave.C  D=Gd_Mwave.D  SampleTime=Control.DT
  Discrete State-Space4 : DiscreteStateSpace  A=InvGp.A  B=InvGp.B  C=InvGp.C  D=InvGp.D  SampleTime=Control.DT
  Gain : Gain  Commented=on  Gain=-Kff_gain
  Gain1 : Gain  Gain=-Kff_gain
  Sum6 : Sum
  FF_CollectivePitch : Outport
  wires:
  Fwave_Surge/1 -> Gain/1
  Gain/1 -> Discrete State-Space/1
  Discrete State-Space1/1 -> Sum6/1
  Discrete State-Space4/1 -> Delay/1
  Gain1/1 -> Discrete State-Space2/1
  Mwave_Pitch/1 -> Gain1/1
  Sum6/1 -> FF_CollectivePitch/1
  Discrete State-Space2/1 -> Discrete State-Space4/1
  Discrete State-Space/1 -> Discrete State-Space1/1
  Delay/1 -> Sum6/2

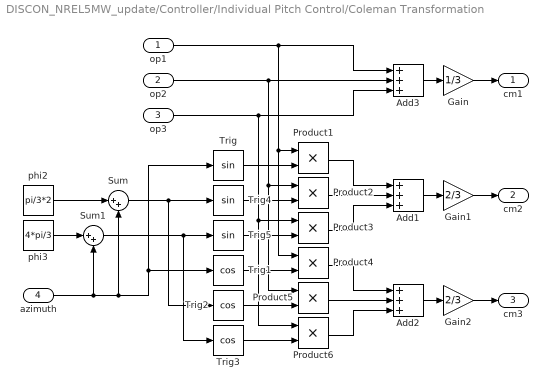
== system DISCON_NREL5MW_update/Controller/Individual Pitch Control/Coleman Transformation ==
  op1 : Inport
  op2 : Inport  Port=2
  op3 : Inport  Port=3
  azimuth : Inport  Port=4
  Add1 : Sum  Inputs=+++
  Add2 : Sum  Inputs=+++
  Add3 : Sum  Inputs=+++
  Gain : Gain  Gain=1/3
  Gain1 : Gain  Gain=2/3
  Gain2 : Gain  Gain=2/3
  Product{1..6} (6 alike) : Product  RndMeth=Zero
  Sum : Sum  Inputs=|++
  Sum1 : Sum  Inputs=|++
  Trig : Trigonometry
  Trig1 : Trigonometry  Operator=cos
  Trig2 : Trigonometry  Operator=cos
  Trig3 : Trigonometry  Operator=cos
  Trig4 : Trigonometry
  Trig5 : Trigonometry
  phi2 : Constant  Value=pi/3*2
  phi3 : Constant  Value=4*pi/3
  cm1 : Outport
  cm2 : Outport  Port=2
  cm3 : Outport  Port=3
  wires:
  Add1/1 -> Gain1/1
  phi2/1 -> Sum/1
  phi3/1 -> Sum1/1
  azimuth/1 -> Sum1/2, Sum/2, Trig/1, Trig1/1
  Trig/1 -> Product1/2
  Trig4/1 -> Product2/2
  Trig5/1 -> Product3/2
  Trig1/1 -> Product4/2
  Trig2/1 -> Product5/2
  Trig3/1 -> Product6/2
  Sum/1 -> Trig4/1, Trig2/1
  Sum1/1 -> Trig5/1, Trig3/1
  Add2/1 -> Gain2/1
  Add3/1 -> Gain/1
  Gain/1 -> cm1/1
  Gain1/1 -> cm2/1
  Gain2/1 -> cm3/1
  op1/1 -> Add3/1, Product1/1, Product4/1
  op2/1 -> Add3/2, Product2/1, Product5/1
  op3/1 -> Add3/3, Product6/1, Product3/1
  Product1/1 -> Add1/1
  Product2/1 -> Add1/2
  Product3/1 -> Add1/3
  Product4/1 -> Add2/1
  Product5/1 -> Add2/2
  Product6/1 -> Add2/3

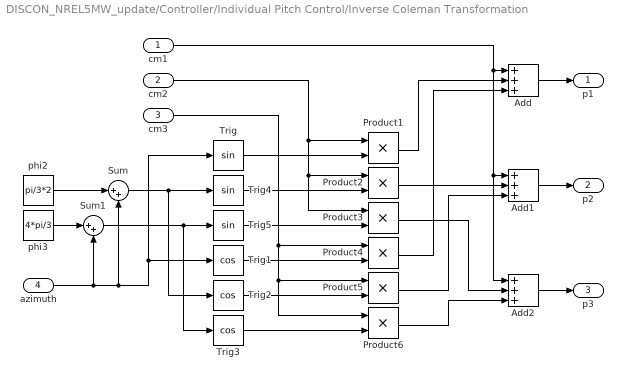
== system DISCON_NREL5MW_update/Controller/Individual Pitch Control/Inverse Coleman Transformation ==
  cm1 : Inport
  cm2 : Inport  Port=2
  cm3 : Inport  Port=3
  azimuth : Inport  Port=4
  Add : Sum  Inputs=+++
  Add1 : Sum  Inputs=+++
  Add2 : Sum  Inputs=+++
  Product{1..6} (6 alike) : Product  RndMeth=Zero
  Sum : Sum  Inputs=|++
  Sum1 : Sum  Inputs=|++
  Trig : Trigonometry
  Trig1 : Trigonometry  Operator=cos
  Trig2 : Trigonometry  Operator=cos
  Trig3 : Trigonometry  Operator=cos
  Trig4 : Trigonometry
  Trig5 : Trigonometry
  phi2 : Constant  Value=pi/3*2
  phi3 : Constant  Value=4*pi/3
  p1 : Outport
  p2 : Outport  Port=2
  p3 : Outport  Port=3
  wires:
  phi2/1 -> Sum/1
  phi3/1 -> Sum1/1
  azimuth/1 -> Sum1/2, Sum/2, Trig/1, Trig1/1
  Sum/1 -> Trig4/1, Trig2/1
  Sum1/1 -> Trig5/1, Trig3/1
  Add/1 -> p1/1
  Add1/1 -> p2/1
  Add2/1 -> p3/1
  Trig/1 -> Product1/2
  Trig4/1 -> Product2/2
  Trig5/1 -> Product3/2
  Trig1/1 -> Product4/2
  Trig2/1 -> Product5/2
  Trig3/1 -> Product6/2
  cm1/1 -> Add/1, Add1/1, Add2/1
  cm2/1 -> Product1/1, Product2/1, Product3/1
  Product1/1 -> Add/2
  Product2/1 -> Add1/2
  Product3/1 -> Add2/2
  cm3/1 -> Product4/1, Product5/1, Product6/1
  Product4/1 -> Add/3
  Product5/1 -> Add1/3
  Product6/1 -> Add2/3

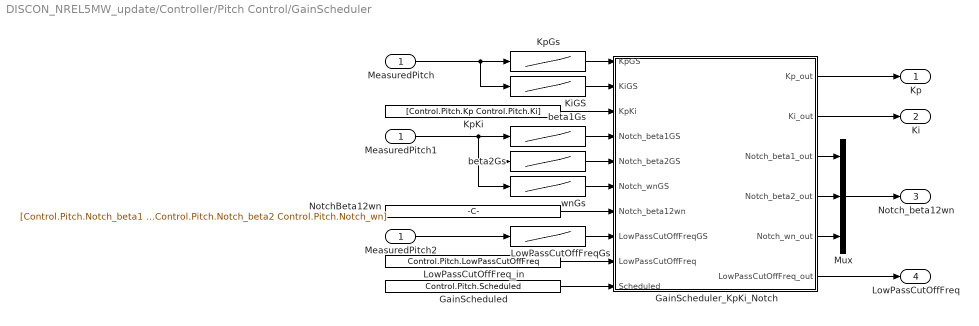
== system DISCON_NREL5MW_update/Controller/Pitch Control/GainScheduler ==
  MeasuredPitch : Inport
  GainScheduled : Constant  Value=Control.Pitch.Scheduled
  GainScheduler_KpKi_Notch : MATLAB Function  TreatAsAtomicUnit=on
  KiGS : Lookup_n-D  NumberOfTableDimensions=1  BreakpointsForDimension1=Control.Pitch.ScheduledPitchAngles  Table=Control.Pitch.KiGS  ExtrapMethod=Clip  UseLastTableValue=on  InternalRulePriority=Speed  RndMeth=Simplest  InputSameDT=on
  KpGs : Lookup_n-D  NumberOfTableDimensions=1  BreakpointsForDimension1=Control.Pitch.ScheduledPitchAngles  Table=Control.Pitch.KpGS  ExtrapMethod=Clip  UseLastTableValue=on  InternalRulePriority=Speed  RndMeth=Simplest  InputSameDT=on
  KpKi : Constant  Value=[Control.Pitch.Kp Control.Pitch.Ki]
  LowPassCutOffFreqGs : Lookup_n-D  NumberOfTableDimensions=1  BreakpointsForDimension1=Control.Pitch.ScheduledPitchAngles  Table=Control.Pitch.LowPassCutOffFreqGS  ExtrapMethod=Clip  UseLastTableValue=on  InternalRulePriority=Speed  RndMeth=Simplest  InputSameDT=on
  LowPassCutOffFreq_in : Constant  Value=Control.Pitch.LowPassCutOffFreq
  MeasuredPitch1 : InportShadow
  MeasuredPitch2 : InportShadow
  Mux : Mux  Inputs=3
  NotchBeta12wn : Constant  Value=[Control.Pitch.Notch_beta1 Control.Pitch.Notch_beta2 Control.Pitch.Notch_wn]
  beta1Gs : Lookup_n-D  NumberOfTableDimensions=1  BreakpointsForDimension1=Control.Pitch.ScheduledPitchAngles  Table=Control.Pitch.Notch_beta1GS  ExtrapMethod=Clip  UseLastTableValue=on  InternalRulePriority=Speed  RndMeth=Simplest  InputSameDT=on
  beta2Gs : Lookup_n-D  NumberOfTableDimensions=1  BreakpointsForDimension1=Control.Pitch.ScheduledPitchAngles  Table=Control.Pitch.Notch_beta2GS  ExtrapMethod=Clip  UseLastTableValue=on  InternalRulePriority=Speed  RndMeth=Simplest  InputSameDT=on
  wnGs : Lookup_n-D  NumberOfTableDimensions=1  BreakpointsForDimension1=Control.Pitch.ScheduledPitchAngles  Table=Control.Pitch.Notch_wnGS  ExtrapMethod=Clip  UseLastTableValue=on  InternalRulePriority=Speed  RndMeth=Simplest  InputSameDT=on
  Kp : Outport  VectorParamsAs1DForOutWhenUnconnected=off
  Ki : Outport  Port=2  VectorParamsAs1DForOutWhenUnconnected=off
  Notch_beta12wn : Outport  Port=3  VectorParamsAs1DForOutWhenUnconnected=off
  LowPassCutOffFreq : Outport  Port=4  VectorParamsAs1DForOutWhenUnconnected=off
  wires:
  MeasuredPitch/1 -> KiGS/1, KpGs/1
  GainScheduled/1 -> GainScheduler_KpKi_Notch/10(Scheduled)
  GainScheduler_KpKi_Notch/2(Ki_out) -> Ki/1
  KpKi/1 -> GainScheduler_KpKi_Notch/3(KpKi)
  KpGs/1 -> GainScheduler_KpKi_Notch/1(KpGS)
  KiGS/1 -> GainScheduler_KpKi_Notch/2(KiGS)
  GainScheduler_KpKi_Notch/1(Kp_out) -> Kp/1
  GainScheduler_KpKi_Notch/3(Notch_beta1_out) -> Mux/1
  GainScheduler_KpKi_Notch/4(Notch_beta2_out) -> Mux/2
  GainScheduler_KpKi_Notch/5(Notch_wn_out) -> Mux/3
  NotchBeta12wn/1 -> GainScheduler_KpKi_Notch/7(Notch_beta12wn)
  MeasuredPitch1/1 -> wnGs/1, beta2Gs/1, beta1Gs/1
  beta1Gs/1 -> GainScheduler_KpKi_Notch/4(Notch_beta1GS)
  beta2Gs/1 -> GainScheduler_KpKi_Notch/5(Notch_beta2GS)
  wnGs/1 -> GainScheduler_KpKi_Notch/6(Notch_wnGS)
  Mux/1 -> Notch_beta12wn/1
  MeasuredPitch2/1 -> LowPassCutOffFreqGs/1
  LowPassCutOffFreqGs/1 -> GainScheduler_KpKi_Notch/8(LowPassCutOffFreqGS)
  LowPassCutOffFreq_in/1 -> GainScheduler_KpKi_Notch/9(LowPassCutOffFreq)
  GainScheduler_KpKi_Notch/6(LowPassCutOffFreq_out) -> LowPassCutOffFreq/1

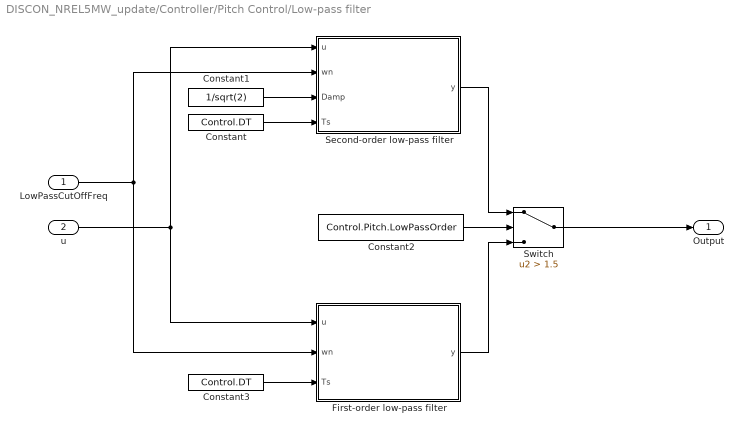
== system DISCON_NREL5MW_update/Controller/Pitch Control/Low-pass filter ==
  LowPassCutOffFreq : Inport
  u : Inport  Port=2
  Constant : Constant  Value=Control.DT
  Constant1 : Constant  Value=1/sqrt(2)
  Constant2 : Constant  Value=Control.Pitch.LowPassOrder
  Constant3 : Constant  Value=Control.DT
  First-order low-pass filter : MATLAB Function  TreatAsAtomicUnit=on
  Second-order low-pass filter : MATLAB Function  TreatAsAtomicUnit=on
  Switch : Switch  Criteria=u2 > Threshold  Threshold=1.5
  Output : Outport  VectorParamsAs1DForOutWhenUnconnected=off
  wires:
  Switch/1 -> Output/1
  Constant1/1 -> Second-order low-pass filter/3(Damp)
  Constant/1 -> Second-order low-pass filter/4(Ts)
  Constant3/1 -> First-order low-pass filter/3(Ts)
  Constant2/1 -> Switch/2
  First-order low-pass filter/1(y) -> Switch/3
  Second-order low-pass filter/1(y) -> Switch/1
  LowPassCutOffFreq/1 -> Second-order low-pass filter/2(wn), First-order low-pass filter/2(wn)
  u/1 -> First-order low-pass filter/1(u), Second-order low-pass filter/1(u)

== system DISCON_NREL5MW_update/Controller/Pitch Control/Notch filter ==
  u : Inport
  beta12wn : Inport  Port=2
  Constant : Constant  Value=Control.DT
  Demux : Demux  Outputs=3
  MATLAB Function : MATLAB Function  TreatAsAtomicUnit=on
  Out1 : Outport  VectorParamsAs1DForOutWhenUnconnected=off
  wires:
  MATLAB Function/1(y) -> Out1/1
  Demux/1 -> MATLAB Function/2(beta1)
  Demux/2 -> MATLAB Function/3(beta2)
  Demux/3 -> MATLAB Function/4(wn)
  beta12wn/1 -> Demux/1
  u/1 -> MATLAB Function/1(u)
  Constant/1 -> MATLAB Function/5(Ts)

== system DISCON_NREL5MW_update/Controller/Torque Control/Low-pass filter ==
  u : Inport
  Constant1 : Constant  Value=Control.Torque.LowPassCutOffFreq
  Constant3 : Constant  Value=Control.DT
  First-order low-pass filter : MATLAB Function  TreatAsAtomicUnit=on
  Output : Outport  VectorParamsAs1DForOutWhenUnconnected=off
  wires:
  Constant3/1 -> First-order low-pass filter/3(Ts)
  u/1 -> First-order low-pass filter/1(u)
  First-order low-pass filter/1(y) -> Output/1
  Constant1/1 -> First-order low-pass filter/2(wn)

== matlab function DISCON_NREL5MW_update/Controller/Pitch Control/PitchControl ==
  settings: updateMethod=DISCRETE  sampleTime=Control.DT
  data: GeneratorSpeedError input; GeneratorSpeed input; MeasuredTorque input; MeasuredPitch input; BladePitch output; KP input; KI input; MinMaxPitch input; MinMaxPitchRate input; DT input; P_InitAngle input; P_StartupPitch input; GearboxRatio input; P_StartUpSpeed input; P_StartupPitchRate input; omega_C input; Demanded_torque input; Clock input; P_LowRateModeOut output boolean; Event input; EventTime input
function [BladePitch, P_LowRateModeOut]  = PitchControl(GeneratorSpeedError, GeneratorSpeed, MeasuredTorque, MeasuredPitch, KP, KI, MinMaxPitch, MinMaxPitchRate, DT, P_InitAngle, P_StartupPitch, GearboxRatio, P_StartUpSpeed, P_StartupPitchRate, omega_C, Demanded_torque, Clock, Event, EventTime)
persistent I_term PI_term_old P_LowRateMode P_LowRateMode_old

%Initialize all persistent variables
if isempty(I_term)
    I_term = 0;
    PI_term_old = 0;
    P_LowRateMode = true;
    P_LowRateMode_old = true; %Used to detect change from start-up/below-rated to above-rated operation mode
    BladePitch=0;
    PitchRate=0;
end

%Event handling part
if (Event == 2 && Clock >= EventTime) || (Event == 5 && Clock >= EventTime) %Grid loss, emergency shutdown
    P_LowRateMode = false;
    P_MinPitchSat = MinMaxPitch(2)*pi/180;
elseif (Event == 4 && Clock >= EventTime) % Normal shutdown
    P_LowRateMode = true;
    P_MinPitchSat = MinMaxPitch(2)*pi/180;
elseif Event == 7 || Event == 6 % Idling and parked mode
    P_MinPitchSat = MinMaxPitch(2)*pi/180;
elseif MeasuredTorque > Demanded_torque*0.99 || GeneratorSpeed > omega_C*(pi/30) % Above-rated operating mode
    P_LowRateMode = false;
    P_MinPitchSat = MinMaxPitch(1)*pi/180;
    if P_LowRateMode ~= P_LowRateMode_old % On switching event between below-rated to above rated, reinitialize the integral term to ensure smooth transition
        I_term = MeasuredPitch;
    end
elseif Event == 3 || GeneratorSpeed < P_StartUpSpeed*GearboxRatio*(pi/30) % Normal startup 
    if Event == 3 && Clock < EventTime
        P_LowRateMode = true;
        P_MinPitchSat = MinMaxPitch(2)*pi/180;
    elseif (Event == 3 && Clock >= EventTime) && (GeneratorSpeed < P_StartUpSpeed*GearboxRatio*(pi/30))
        P_LowRateMode = true;
        P_MinPitchSat = P_StartupPitch*pi/180;
    else
        P_LowRateMode = true;
        P_MinPitchSat = MinMaxPitch(1)*pi/180;
    end
else
    P_MinPitchSat = MinMaxPitch(1)*pi/180;
end
 
% Pitch controller, KP and KI are constant or gain-scheduled, depending on
% input. Integral term is saturated, lower bound is variable and depends on
% event or operatinig mode.
P_term = KP*GeneratorSpeedError;
I_term = I_term + KI*GeneratorSpeedError*DT;
I_term = min(max(I_term,P_MinPitchSat), MinMaxPitch(2)*pi/180);

PI_term = P_term + I_term;
PI_term_sat = min(max(PI_term,P_MinPitchSat), MinMaxPitch(2)*pi/180);

% Calculate and limit pitch rate. Limit on rate is subject to event or
% operating mode.
PitchRate = (PI_term_sat - PI_term_old)/DT;
if P_LowRateMode
    PitchRate = min(max(PitchRate, -P_StartupPitchRate*pi/180), P_StartupPitchRate*pi/180);
else
    PitchRate = min(max(PitchRate, MinMaxPitchRate(1)*pi/180), MinMaxPitchRate(2)*pi/180);
end
BladePitch = PI_term_old + PitchRate*DT;

% Write variables to persistent variables and/or outputs
PI_term_old = BladePitch;
P_LowRateModeOut = P_LowRateMode;
P_LowRateMode_old = P_LowRateMode;
end

== matlab function DISCON_NREL5MW_update/Controller/Pitch Control/GainScheduler/GainScheduler_KpKi_Notch ==
  data: KpGS input; KiGS input; Kp_out output; KpKi input; Notch_beta1GS input; Notch_beta2GS input; Notch_wnGS input; Notch_beta12wn input; LowPassCutOffFreqGS input; LowPassCutOffFreq input; Scheduled input; Ki_out output; Notch_beta1_out output; Notch_beta2_out output; Notch_wn_out output; LowPassCutOffFreq_out output
function [Kp_out, Ki_out, Notch_beta1_out, Notch_beta2_out, Notch_wn_out, LowPassCutOffFreq_out] = fcn(KpGS, KiGS, KpKi, Notch_beta1GS, Notch_beta2GS, Notch_wnGS, Notch_beta12wn, LowPassCutOffFreqGS, LowPassCutOffFreq, Scheduled)

if Scheduled > 0.5
    Kp_out = KpGS;
    Ki_out = KiGS;
    Notch_beta1_out = Notch_beta1GS;
    Notch_beta2_out = Notch_beta2GS;
    Notch_wn_out = Notch_wnGS;
    LowPassCutOffFreq_out = LowPassCutOffFreqGS;
else
    Kp_out = KpKi(1);
    Ki_out = KpKi(2);
    Notch_beta1_out = Notch_beta12wn(1);
    Notch_beta2_out = Notch_beta12wn(2);
    Notch_wn_out = Notch_beta12wn(3);
    LowPassCutOffFreq_out = LowPassCutOffFreq;
end

== matlab function DISCON_NREL5MW_update/Controller/Pitch Control/Notch filter/MATLAB Function ==
  data: u input; beta1 input; beta2 input; wn input; y output; Ts input
function y = NotchFilter(u, beta1, beta2, wn, Ts)

persistent u_prev1 u_prev2 y_prev1 y_prev2
if isempty(u_prev1)
    u_prev1 = u;
    u_prev2 = u;
    y_prev1 = u;
    y_prev2 = u;
    y=0;
end

if any([beta1 beta2 wn] == 0)
    y = u;
else
    % Prepare filter elements from current input
    K = 2/Ts;
    Part1 = (K^2 + 2*wn*beta1 * K + wn^2) / (K^2 + 2*wn*beta2 * K + wn^2);
    Part2 = (2 * wn^2 - 2 * K^2)  / (K^2 + 2*wn*beta2 * K + wn^2);
    Part3 = (K^2 - 2*wn*beta1 * K + wn^2) / (K^2 + 2*wn*beta2 * K + wn^2);
    Part4 = (2 * wn^2 - 2 * K^2)  / (K^2 + 2*wn*beta2 * K + wn^2);
    Part5 = (K^2 - 2*wn*beta2* K + wn^2)/ (K^2 + 2*wn*beta2 * K + wn^2);
    
    % Compute filter output
    y = Part1*u + Part2*u_prev1 + Part3*u_prev2 - Part4*y_prev1 - Part5*y_prev2;
    
    % Save signals for next time step
    u_prev2 = u_prev1;
    u_prev1 = u;
    
    y_prev2 = y_prev1;
    y_prev1 = y;
end

== matlab function DISCON_NREL5MW_update/Controller/Pitch Control/Low-pass filter/Second-order low-pass filter ==
  data: u input; wn input; Damp input; y output; Ts input
function y = SecLPF(u, wn, Damp, Ts)

persistent y_prev1 y_prev2 u_prev1 u_prev2

if isempty(u_prev1)
    y_prev1 = u;
    y_prev2 = u;
    u_prev1 = u;
    u_prev2 = u;
    y=0;
end

y = 1/(4+4*Ts*Damp*wn+Ts^2*wn^2) * ( (8-2*Ts^2*wn^2)*y_prev1 + ...
    (-4+4*Ts*Damp*wn-Ts^2*wn^2)*y_prev2 + (Ts^2*wn^2)*u ...
    + (2*Ts^2*wn^2)*u_prev1 + (Ts^2*wn^2)*u_prev2 );

u_prev2   = u_prev1;
u_prev1   = u;
y_prev2  = y_prev1;
y_prev1  = y;

== matlab function DISCON_NREL5MW_update/Controller/Pitch Control/Low-pass filter/First-order low-pass filter ==
  data: u input; wn input; y output; Ts input
function y = FirstLPF(u, wn, Ts)

persistent y_prev1 u_prev1

if isempty(u_prev1)
    y_prev1 = u;
    u_prev1 = u;
end

y = (Ts*wn*u + Ts*wn*u_prev1 - (Ts*wn-2.0)*y_prev1)/(Ts*wn+2.0);

u_prev1   = u;
y_prev1  = y;

== matlab function DISCON_NREL5MW_update/Controller/Torque Control/Low-pass filter/First-order low-pass filter ==
  data: u input; wn input; y output; Ts input
function y = FirstLPF(u, wn, Ts)

persistent y_prev1 u_prev1

if isempty(u_prev1)
    y_prev1 = u;
    u_prev1 = u;
end

y = (Ts*wn*u + Ts*wn*u_prev1 - (Ts*wn-2.0)*y_prev1)/(Ts*wn+2.0);

u_prev1   = u;
y_prev1  = y;

== matlab function DISCON_NREL5MW_update/Controller/Pitch_Saturation_2/Rate Saturation Pitch ==
  data: u input; MinSaturation input; y_out output size=1; MaxSaturation input; DT input
function y_out = fcn(u, MinSaturation, MaxSaturation, DT)
persistent y2

if isempty(y2)
    y2 = u;
end

rate = (u-y2)/DT;
rate = min(max(rate, MinSaturation), MaxSaturation);

y2 = y2 + rate*DT;
y_out = y2;

== matlab function DISCON_NREL5MW_update/Controller/Pitch_Saturation_3/Rate Saturation Pitch ==
  data: u input; MinSaturation input; y_out output; MaxSaturation input; DT input
function y_out = fcn(u, MinSaturation, MaxSaturation, DT)
persistent y

if isempty(y)
    y = u;
    yout=0;
end

rate = (u-y)/DT;
rate = min(max(rate, MinSaturation), MaxSaturation);

y = y + rate*DT;
y_out = y;

== matlab function DISCON_NREL5MW_update/Controller/Collective_Pitch_Saturation/Rate Saturation Pitch ==
  data: u input; MinSaturation input; y_out output size=1; MaxSaturation input; DT input
function y_out = fcn(u, MinSaturation, MaxSaturation, DT)
persistent y

if isempty(y)
    y = u;
end

rate = (u-y)/DT;
rate = min(max(rate, MinSaturation), MaxSaturation);

y = y + rate*DT;
y_out = y;

== matlab function DISCON_NREL5MW_update/Controller/Subsystem/Tower Fore-Aft Control ==
  data: Rel_WindVelocity input; AddBladePitch output; TwrFA_Velocity input; AddGenTorque output; K_TFABPD input; K_TFAGTD input; K_BPD output; K_GTD output
function [AddBladePitch,AddGenTorque,K_BPD,K_GTD] = TowerForeAft(Rel_WindVelocity,TwrFA_Velocity, K_TFABPD, K_TFAGTD)

persistent AddBladePitchAngle GenTorqueAdded K_TFA_Damp K_TFA_RHPZComp

%Initialize all persistent variables
if isempty(AddBladePitchAngle)
    AddBladePitchAngle = 0;
    GenTorqueAdded = 0;
    K_TFA_Damp = 0;
    K_TFA_RHPZComp = 0;
end

Vinf_BelowRated = (0:10);
Vinf_op = [Vinf_BelowRated,11.4,12:1:25];

%% Tower Damping via Collective Blade Pitch
% Here the tower-top acceleration/velocity is fed back to the Blade Pitch
K_TFA_Damp = interp1(Vinf_op,K_TFABPD,Rel_WindVelocity);
%P_MinPitchSat = FinePitchAngle*pi/180;                       % Minimum blade pitch (rad) 

AddBladePitchAngle = K_TFA_Damp*TwrFA_Velocity*(pi/180);      % rad
AddBladePitch = AddBladePitchAngle;
K_BPD = K_TFA_Damp;

%% RHPZ compensation
% Here the tower-top acceleration/velocity is fed back to the generator torque
K_TFA_RHPZComp = interp1(Vinf_op,K_TFAGTD,Rel_WindVelocity);
GenTorqueAdded = K_TFA_RHPZComp*TwrFA_Velocity;
AddGenTorque = GenTorqueAdded;
K_GTD = K_TFA_RHPZComp;

== matlab function DISCON_NREL5MW_update/Controller/Generator Torque Rate Saturation/Rate Saturation Torque ==
  data: u input; MinSaturation input; y_out output; MaxSaturation input; DT input
function y_out = fcn(u, MinSaturation, MaxSaturation, DT)
persistent y

if isempty(y)
    y = u;
end

rate = (u-y)/DT;
rate = min(max(rate, MinSaturation), MaxSaturation);

y = y + rate*DT;
y_out = y;

== matlab function DISCON_NREL5MW_update/Controller/Pitch_Saturation_1/Rate Saturation Pitch ==
  data: u input; MinSaturation input; y_out output size=1; MaxSaturation input; DT input
function y_out = fcn(u, MinSaturation, MaxSaturation, DT)
persistent y

if isempty(y)
    y = u;
end

rate = (u-y)/DT;
rate = min(max(rate, MinSaturation), MaxSaturation);

y = y + rate*DT;
y_out = y;

== matlab function DISCON_NREL5MW_update/Controller/Torque Control/TorqueController ==
  data: GeneratorTorqueDemand output; MeasuredGeneratorSpeed input; MeasuredPitch input; Control_Torque_OptGain input; omega_ABCD input size=[1 4]; P_StartupMode input; Torque_Demanded input; FineMaxPitch input; T_MinTorque input; Clock input; Event input; EventTime input
function GeneratorTorqueDemand  = TorqueController(MeasuredGeneratorSpeed, MeasuredPitch, Control_Torque_OptGain, omega_ABCD, P_StartupMode, Torque_Demanded, FineMaxPitch, T_MinTorque, Clock, Event, EventTime)

% Calculate generator torque setpoint according to the feedforward wind
% turbine control law T = K*\omega^2
GeneratorTorqueDemand = max(min(Control_Torque_OptGain*MeasuredGeneratorSpeed^2, Torque_Demanded), T_MinTorque);

% Calculate torques at beginning and end of CP_max operation
TorqueOmegaB = Control_Torque_OptGain*(omega_ABCD(2)*pi/30)^2;
TorqueOmegaC = Control_Torque_OptGain*(omega_ABCD(3)*pi/30)^2;

% Apply maximum demanded torque when pitch is 1 degree above fine-pitch and
% the wind turbine is not in start-up mode.
if (Event == 5 && Clock >= EventTime) && (MeasuredPitch > (FineMaxPitch(2) - 1.0)*pi/180) %Emergency shutdown
    GeneratorTorqueDemand = 0.0;
elseif MeasuredPitch > (FineMaxPitch(1) + 1.0)*pi/180 && P_StartupMode == false
    GeneratorTorqueDemand = Torque_Demanded;
elseif MeasuredGeneratorSpeed < omega_ABCD(1)*pi/30
    GeneratorTorqueDemand = T_MinTorque;
elseif MeasuredGeneratorSpeed < omega_ABCD(2)*pi/30
    GeneratorTorqueDemand = (TorqueOmegaB - T_MinTorque)/((omega_ABCD(2) - omega_ABCD(1))*pi/30)*(MeasuredGeneratorSpeed - omega_ABCD(1)*pi/30) + T_MinTorque;
elseif MeasuredGeneratorSpeed >= omega_ABCD(3)*pi/30
    GeneratorTorqueDemand = (Torque_Demanded - TorqueOmegaC)/((omega_ABCD(4) - omega_ABCD(3))*pi/30)*(MeasuredGeneratorSpeed - omega_ABCD(3)*pi/30) + TorqueOmegaC;
end
